simulink model "consulta_sistema_base"  (R2023a)
settings: Solver=VariableStepAuto  StartTime=0.0  StopTime=2  RelTol=1e-3
values from neighbouring files (symbols this model uses):
  filtros = banco_decodificador(Fs, frecuencias_centrales, orden)    [main.m]    (also in sim_falla.m; sim_ideal.m; sim_real.m)
  Fs = 44000    [butter_digital_frec_resp.m]    (also in canal.m; main.m; sim_falla.m; sim_ideal.m)
undefined symbols (not defined in the file or in its folder): f_canal_den, f_canal_num, f_portadora_den, f_portadora_num
libraries: dspstat3 x2
settings Model: Creator=mluser  LastModifiedBy=lcampero

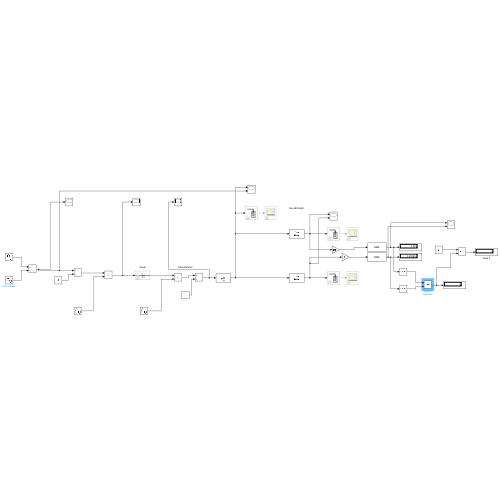
[thumbnail: Simulink's stored preview of the top-level diagram]
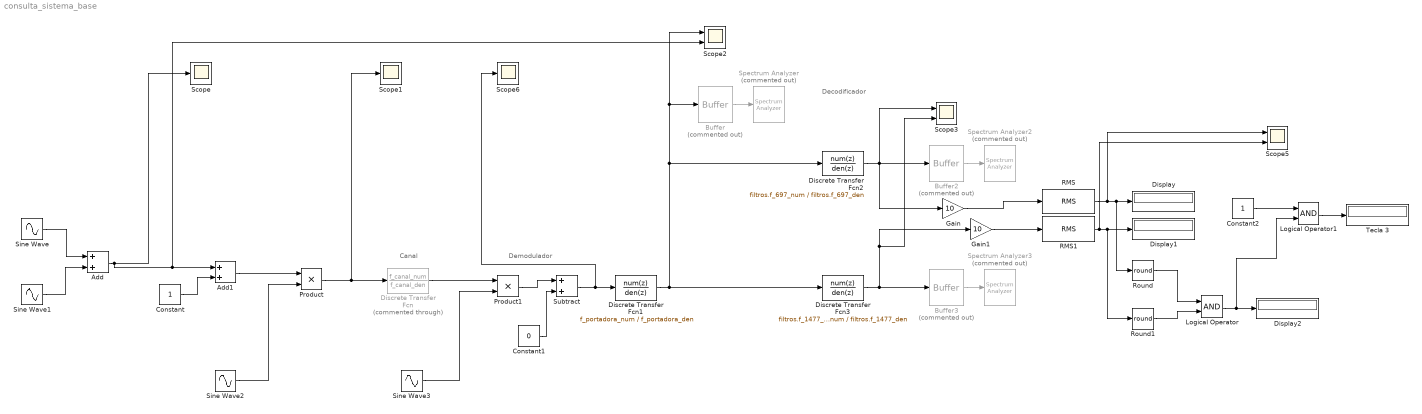
== system consulta_sistema_base ==
  note: Decodificador
  note: Canal
  note: Demodulador
  Add : Sum
  Add1 : Sum
  Buffer : Buffer  Commented=on  N=1024  OutputFrames=off
  Buffer2 : Buffer  Commented=on  N=1024  OutputFrames=off
  Buffer3 : Buffer  Commented=on  N=1024  OutputFrames=off
  Constant : Constant
  Constant1 : Constant  Value=0
  Constant2 : Constant
  Discrete Transfer Fcn : DiscreteTransferFcn  Commented=through  Numerator=f_canal_num  Denominator=f_canal_den  SampleTime=1/Fs
  Discrete Transfer Fcn1 : DiscreteTransferFcn  Numerator=f_portadora_num  Denominator=f_portadora_den  SampleTime=1/Fs
  Discrete Transfer Fcn2 : DiscreteTransferFcn  Numerator=filtros.f_697_num  Denominator=filtros.f_697_den  SampleTime=1/Fs
  Discrete Transfer Fcn3 : DiscreteTransferFcn  Numerator=filtros.f_1477_num  Denominator=filtros.f_1477_den  SampleTime=1/Fs
  Display : Display
  Display1 : Display
  Display2 : Display
  Gain : Gain  Gain=10
  Gain1 : Gain  Gain=10
  Logical Operator : Logic  AllPortsSameDT=off  OutDataTypeStr=boolean
  Logical Operator1 : Logic  AllPortsSameDT=off  OutDataTypeStr=boolean
  Product : Product
  Product1 : Product
  RMS : dspstat3/RMS  run=off  directionMode=Each column  dimension=1  InputProcessing=Columns as channels (frame based)  reset_popup=None
  RMS1 : dspstat3/RMS  run=off  directionMode=Each column  dimension=1  InputProcessing=Columns as channels (frame based)  reset_popup=None
  Round : Rounding  Operator=round
  Round1 : Rounding  Operator=round
  Scope : Scope
  Scope1 : Scope
  Scope2 : Scope  NumInputPorts=2
  Scope3 : Scope  NumInputPorts=2
  Scope5 : Scope  NumInputPorts=2
  Scope6 : Scope
  Sine Wave : Sin  Amplitude=0.3  Frequency=2*pi*697  SampleTime=1/Fs
  Sine Wave1 : Sin  Amplitude=0.3  Frequency=2*pi*1209  SampleTime=1/Fs
  Sine Wave2 : Sin  Frequency=2*pi*15000  SampleTime=1/Fs
  Sine Wave3 : Sin  Frequency=2*pi*15000  SampleTime=1/Fs
  Spectrum Analyzer : SpectrumAnalyzer  Commented=on  WindowPosition=[1.000000,1.000000,1920.000000,1016.000000,]  ScopeFrameLocation=window  SampleRateSource=Property  SampleRate=44.1e3  PlotAsTwoSidedSpectrum=off  FrequencyScale=Log  FrequencySpan=Start and stop frequencies  StartFrequency=20  StopFrequency=20e3  YLimits=[-268.71750201,55.58512554]  ColorLimits=[-20 80]  DefaultConfigurationName=spbscopes.SpectrumAnalyzerBlockCfg  IsFrequencyInputMode=0  FrequencyVectorPort=0  FrequencyVectorFromPort=0  FrequencyInputRBWPort=0  FrequencyInputRBWFromPort=0
  Spectrum Analyzer2 : SpectrumAnalyzer  Commented=on  WindowPosition=[948.000000,212.000000,973.000000,545.000000,]  ScopeFrameLocation=window  SampleRateSource=Property  SampleRate=44.1e3  PlotAsTwoSidedSpectrum=off  FrequencyScale=Log  FrequencySpan=Start and stop frequencies  StartFrequency=20  StopFrequency=20e3  YLimits=[-283.95090686,42.27775884]  ColorLimits=[-20 80]  DefaultConfigurationName=spbscopes.SpectrumAnalyzerBlockCfg  IsFrequencyInputMode=0  FrequencyVectorPort=0  FrequencyVectorFromPort=0  FrequencyInputRBWPort=0  FrequencyInputRBWFromPort=0
  Spectrum Analyzer3 : SpectrumAnalyzer  Commented=on  WindowPosition=[1.000000,195.000000,964.000000,558.000000,]  ScopeFrameLocation=window  SampleRateSource=Property  SampleRate=44.1e3  PlotAsTwoSidedSpectrum=off  FrequencyScale=Log  FrequencySpan=Start and stop frequencies  StartFrequency=20  StopFrequency=20e3  YLimits=[-286.78350788,39.68128921]  ColorLimits=[-20 80]  DefaultConfigurationName=spbscopes.SpectrumAnalyzerBlockCfg  IsFrequencyInputMode=0  FrequencyVectorPort=0  FrequencyVectorFromPort=0  FrequencyInputRBWPort=0  FrequencyInputRBWFromPort=0
  Subtract : Sum
  Tecla 3 : Display
  wires:
  Sine Wave/1 -> Add/1
  Sine Wave1/1 -> Add/2
  Add/1 -> Scope2/2, Add1/1, Scope/1
  Constant/1 -> Add1/2
  Add1/1 -> Product/1
  Sine Wave2/1 -> Product/2
  Product/1 -> Scope1/1, Discrete Transfer Fcn/1
  Sine Wave3/1 -> Product1/2
  Discrete Transfer Fcn1/1 -> Discrete Transfer Fcn3/1, Discrete Transfer Fcn2/1, Scope2/1, Buffer/1
  Buffer/1 -> Spectrum Analyzer/1
  Product1/1 -> Subtract/1
  Buffer2/1 -> Spectrum Analyzer2/1
  Discrete Transfer Fcn2/1 -> Gain/1, Scope3/1, Buffer2/1
  Buffer3/1 -> Spectrum Analyzer3/1
  Discrete Transfer Fcn/1 -> Product1/1
  Subtract/1 -> Scope6/1, Discrete Transfer Fcn1/1
  Constant1/1 -> Subtract/2
  RMS/1 -> Scope5/1, Round/1, Display/1
  RMS1/1 -> Scope5/2, Round1/1, Display1/1
  Discrete Transfer Fcn3/1 -> Scope3/2, Gain1/1, Buffer3/1
  Gain/1 -> RMS/1
  Gain1/1 -> RMS1/1
  Logical Operator/1 -> Logical Operator1/2, Display2/1
  Round/1 -> Logical Operator/1
  Round1/1 -> Logical Operator/2
  Constant2/1 -> Logical Operator1/1
  Logical Operator1/1 -> Tecla 3/1
